simulink model "SolarInverter_DigitalTwin"  (R2019b)
settings: Solver=ode23tb  StartTime=0.0  StopTime=inf  RelTol=1e-3
InitFcn:
  | SolarInverter_Params();
values from neighbouring files (symbols this model uses):
  Fnom = 60    [SolarInverter_Params.m]
  Pnom = 112e3    (= 112000)    [SolarInverter_Params.m]
  reec_dbd1 = -0.1    [SolarInverter_Params.m]
  reec_dbd2 = 0.1    [SolarInverter_Params.m]
  reec_dPmax = 0.1    [SolarInverter_Params.m]
  reec_dPmin = -0.1    [SolarInverter_Params.m]
  reec_Imax = 1    [SolarInverter_Params.m]
  reec_Iqhl = 1.0    (= 1)    [SolarInverter_Params.m]
  reec_Iqll = -0.4    [SolarInverter_Params.m]
  reec_Kqi = 0.0    (= 0)    [SolarInverter_Params.m]
  reec_Kqp = 0    [SolarInverter_Params.m]
  reec_Kvi = 0.0    (= 0)    [SolarInverter_Params.m]
  reec_Kvp = 0.1    [SolarInverter_Params.m]
  reec_Pmax = 1.0    (= 1)    [SolarInverter_Params.m]
  reec_Pmin = 0    [SolarInverter_Params.m]
  reec_Qmax = 0.435    [SolarInverter_Params.m]
  reec_Qmin = -0.435    [SolarInverter_Params.m]
  reec_Tiq = 0.02    [SolarInverter_Params.m]
  reec_Tp = 0.02    [SolarInverter_Params.m]
  reec_Tpord = 0.1    [SolarInverter_Params.m]
  reec_Trv = 0.01    [SolarInverter_Params.m]
  reec_Vdip = 0.9    [SolarInverter_Params.m]
  reec_Vmax = 1.10    (= 1.1)    [SolarInverter_Params.m]
  reec_Vmin = 0.9    [SolarInverter_Params.m]
  reec_Vup = 1.15    [SolarInverter_Params.m]
  regc_Brkpt = 0.9    [SolarInverter_Params.m]
  regc_Iolim = -1.2    [SolarInverter_Params.m]
  regc_Iqrmax = 999.9    [SolarInverter_Params.m]
  regc_Iqrmin = -999.9    [SolarInverter_Params.m]
  regc_Ivpnt0 = 0.4    [SolarInverter_Params.m]
  regc_Ivpnt1 = 0.8    [SolarInverter_Params.m]
  regc_Khv = 0.0    (= 0)    [SolarInverter_Params.m]
  regc_Lvpl1 = 1.0    (= 1)    [SolarInverter_Params.m]
  regc_Lvplsw = 0    [SolarInverter_Params.m]
  regc_rrpwr = 10    [SolarInverter_Params.m]
  regc_Tfltr = 0.02    [SolarInverter_Params.m]
  regc_Tg = 0.1    [SolarInverter_Params.m]
  regc_Volim = 1.1    [SolarInverter_Params.m]
  regc_Zerox = 0.5    [SolarInverter_Params.m]
  repc_db1 = 0    [SolarInverter_Params.m]
  repc_Ddn = 20    [SolarInverter_Params.m]
  repc_Dup = 0    [SolarInverter_Params.m]
  repc_emax = 999    [SolarInverter_Params.m]
  repc_emin = -999    [SolarInverter_Params.m]
  repc_fdbd1 = 0.01*0    (= 0)    [SolarInverter_Params.m]
  repc_fdbd2 = -0.01*0    (= 0)    [SolarInverter_Params.m]
  repc_femax = 999    [SolarInverter_Params.m]
  repc_femin = -999    [SolarInverter_Params.m]
  repc_Kc = 0.05    [SolarInverter_Params.m]
  repc_Ki = 1.8    [SolarInverter_Params.m]
  repc_Kig = 0.5    [SolarInverter_Params.m]
  repc_Kp = 0.6    [SolarInverter_Params.m]
  repc_Kpg = 0.1    [SolarInverter_Params.m]
  repc_Pmax = 1    [SolarInverter_Params.m]
  repc_Pmin = 0    [SolarInverter_Params.m]
  repc_Qmax = inf    [SolarInverter_Params.m]
  repc_Qmin = -inf    [SolarInverter_Params.m]
  repc_Rc = 0    [SolarInverter_Params.m]
  repc_Tfltr = 0.02    [SolarInverter_Params.m]
  repc_Tft = 0.5    [SolarInverter_Params.m]
  repc_Tfv = 0.8    [SolarInverter_Params.m]
  repc_Tlag = 0.2    [SolarInverter_Params.m]
  repc_Tp = 0.25    [SolarInverter_Params.m]
  repc_Vfrz = 0.7    [SolarInverter_Params.m]
  repc_Xc = 0    [SolarInverter_Params.m]
  Vnom = 142e3    (= 142000)    [SolarInverter_Params.m]
undefined symbols (not defined in the file or in its folder): gcbh, j, sps_rtmsupport
libraries: simulink x15, powerlib x7, powerlib_meascontrol x2
(part 2 of 2)

== system SolarInverter_DigitalTwin/Utility-scale Solar Plant Controller/P Filter ==
  u : Inport
  1/(taus+1) : Subsystem  mask{tau=tau, vmax=vmax, vmin=vmin}
      mask prompts: tau "Time Constant"
  k : Gain  Gain=k
  y : Outport  VectorParamsAs1DForOutWhenUnconnected=off
  wires:
  k/1 -> 1/(taus+1)/1(u)
  u/1 -> k/1
  1/(taus+1)/1(y) -> y/1

== system SolarInverter_DigitalTwin/Utility-scale Solar Plant Controller/Q Filter ==
  u : Inport
  1/(taus+1) : Subsystem  mask{tau=tau, vmax=vmax, vmin=vmin}
      mask prompts: tau "Time Constant"
  k : Gain  Gain=k
  y : Outport  VectorParamsAs1DForOutWhenUnconnected=off
  wires:
  k/1 -> 1/(taus+1)/1(u)
  u/1 -> k/1
  1/(taus+1)/1(y) -> y/1

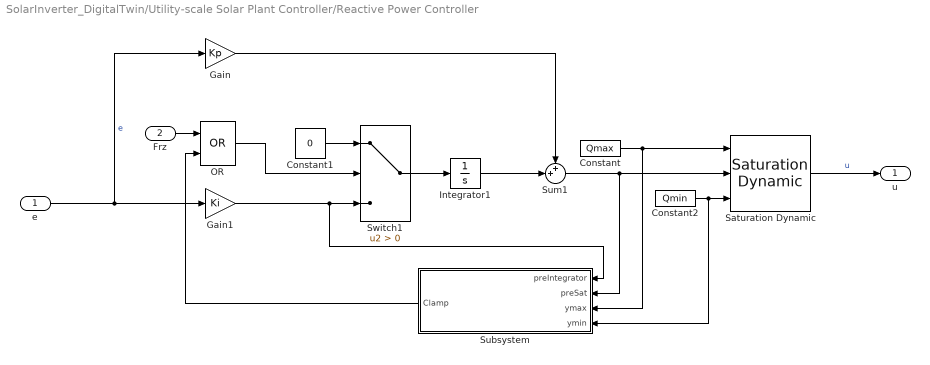
== system SolarInverter_DigitalTwin/Utility-scale Solar Plant Controller/Reactive Power Controller ==
  e : Inport
  Frz : Inport  Port=2
  Constant : Constant  Value=Qmax
  Constant1 : Constant  Value=0
  Constant2 : Constant  Value=Qmin
  Gain : Gain  Gain=Kp
  Gain1 : Gain  Gain=Ki
  Integrator1 : Integrator
  OR : Logic  Operator=OR  AllPortsSameDT=off  OutDataTypeStr=boolean
  Saturation Dynamic : simulink/Discontinuities/Saturation Dynamic  OutMin=[]  OutMax=[]  OutDataTypeStr=Inherit: Same as second input  OutDataType=fixdt(1, 16)  OutScaling=2^-10  DoSatur=off
  Subsystem : Subsystem
  Sum1 : Sum  Inputs=++|
  Switch1 : Switch  Criteria=u2 > Threshold
  u : Outport  VectorParamsAs1DForOutWhenUnconnected=off
  wires:
  OR/1 -> Switch1/2
  Subsystem/1(Clamp) -> OR/2
  Frz/1 -> OR/1
  Constant2/1 -> Saturation Dynamic/3, Subsystem/4(ymin)
  Sum1/1 -> Saturation Dynamic/2, Subsystem/2(preSat)
  Saturation Dynamic/1 -> u/1  "u"
  Switch1/1 -> Integrator1/1
  Gain1/1 -> Switch1/3, Subsystem/1(preIntegrator)
  Integrator1/1 -> Sum1/2
  Constant/1 -> Saturation Dynamic/1, Subsystem/3(ymax)
  Constant1/1 -> Switch1/1
  e/1 -> Gain1/1, Gain/1  "e"
  Gain/1 -> Sum1/1

== system SolarInverter_DigitalTwin/Utility-scale Solar Plant Controller/Subsystem ==
  Ibranch : Inport
  Vreg : Inport  Port=2
  Complex to Magnitude : ComplexToMagnitudeAngle  Output=Magnitude
  Gain : Gain  Gain=Rc
  Gain1 : Gain  Gain=j*Xc
  Sum : Sum  Inputs=|++
  Sum1 : Sum  Inputs=|-+
  Ve : Outport  VectorParamsAs1DForOutWhenUnconnected=off
  wires:
  Ibranch/1 -> Gain/1, Gain1/1
  Gain/1 -> Sum/1
  Vreg/1 -> Sum1/2
  Sum/1 -> Sum1/1
  Gain1/1 -> Sum/2
  Sum1/1 -> Complex to Magnitude/1
  Complex to Magnitude/1 -> Ve/1  "Ve"

== system SolarInverter_DigitalTwin/Utility-scale Solar Plant Controller/Vcomp Filter ==
  u : Inport
  1/(taus+1) : Subsystem  mask{tau=tau, vmax=vmax, vmin=vmin}
      mask prompts: tau "Time Constant"
  k : Gain  Gain=k
  y : Outport  VectorParamsAs1DForOutWhenUnconnected=off
  wires:
  k/1 -> 1/(taus+1)/1(u)
  u/1 -> k/1
  1/(taus+1)/1(y) -> y/1

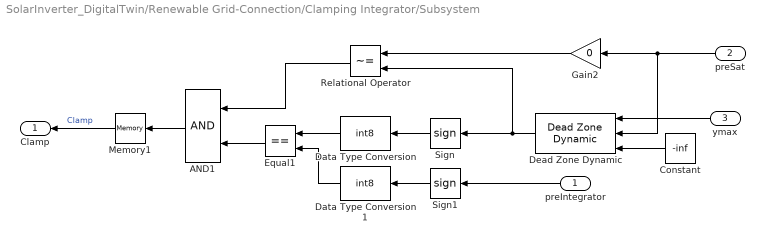
== system SolarInverter_DigitalTwin/Renewable Grid-Connection/Clamping Integrator/Subsystem ==
  preIntegrator : Inport
  preSat : Inport  Port=2
  ymax : Inport  Port=3
  AND1 : Logic  AllPortsSameDT=off  OutDataTypeStr=boolean
  Constant : Constant  Value=-inf
  Data Type Conversion : DataTypeConversion  OutDataTypeStr=int8
  Data Type Conversion1 : DataTypeConversion  OutDataTypeStr=int8
  Dead Zone Dynamic : simulink/Discontinuities/Dead Zone Dynamic
      settings: SourceProductName=Simulink  SourceProductBaseCode=SL
  Equal1 : RelationalOperator  Operator===  OutDataTypeStr=boolean  RndMeth=Simplest
  Gain2 : Gain  Gain=0
  Memory1 : Memory
  Relational Operator : RelationalOperator  Operator=~=  OutDataTypeStr=boolean  RndMeth=Simplest
  Sign : Signum
  Sign1 : Signum
  Clamp : Outport  VectorParamsAs1DForOutWhenUnconnected=off
  wires:
  Sign/1 -> Data Type Conversion/1
  AND1/1 -> Memory1/1
  Dead Zone Dynamic/1 -> Relational Operator/2, Sign/1
  Data Type Conversion/1 -> Equal1/1
  Gain2/1 -> Relational Operator/1
  Equal1/1 -> AND1/2
  preSat/1 -> Dead Zone Dynamic/2, Gain2/1
  Relational Operator/1 -> AND1/1
  Sign1/1 -> Data Type Conversion1/1
  preIntegrator/1 -> Sign1/1
  Data Type Conversion1/1 -> Equal1/2
  ymax/1 -> Dead Zone Dynamic/1
  Constant/1 -> Dead Zone Dynamic/3
  Memory1/1 -> Clamp/1  "Clamp"

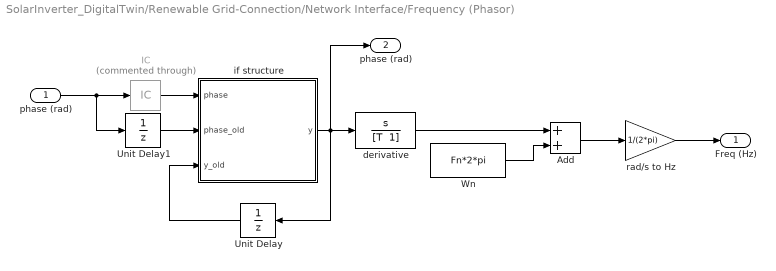
== system SolarInverter_DigitalTwin/Renewable Grid-Connection/Network Interface/Frequency (Phasor) ==
  phase (rad) : Inport
  " Wn" : Constant  Value=Fn*2*pi
  Add : Sum
  IC : InitialCondition  Commented=through  Value=0
  Unit Delay : UnitDelay  SampleTime=-1  HasFrameUpgradeWarning=on
  Unit Delay1 : UnitDelay  SampleTime=-1  HasFrameUpgradeWarning=on
  derivative : TransferFcn  Numerator="[1  0]"  Denominator="[T  1]"
  if structure : MATLAB Function  TreatAsAtomicUnit=on
  rad/s to Hz : Gain  Gain=1/(2*pi)
  Freq (Hz) : Outport  VectorParamsAs1DForOutWhenUnconnected=off
  "phase (rad) " : Outport  Port=2  VectorParamsAs1DForOutWhenUnconnected=off
  wires:
  Add/1 -> rad/s to Hz/1
  if structure/1(y) -> Unit Delay/1, derivative/1, "phase (rad) "/1
  rad/s to Hz/1 -> Freq (Hz)/1
  derivative/1 -> Add/1
  " Wn"/1 -> Add/2
  IC/1 -> if structure/1(phase)
  Unit Delay/1 -> if structure/3(y_old)
  Unit Delay1/1 -> if structure/2(phase_old)
  phase (rad)/1 -> Unit Delay1/1, IC/1

== system SolarInverter_DigitalTwin/Renewable Grid-Connection/Network Interface/Three-phase Interface ==
  Iactive : Inport
  Ireactive : Inport  Port=2
  Controlled Current Source : powerlib/Electrical Sources/Controlled Current Source  Initialize=on  Source_Type=AC  Amplitude=-1*Pnom/sqrt(3)/Vnom*sqrt(2)  Phase=0  Frequency=Fnom  Measurements=None
      settings: SourceProductName=Simscape Electrical
  Controlled Current Source1 : powerlib/Electrical Sources/Controlled Current Source  Initialize=on  Source_Type=AC  Amplitude=-1*Pnom/sqrt(3)/Vnom*sqrt(2)  Phase=120  Frequency=Fnom  Measurements=None
      settings: SourceProductName=Simscape Electrical
  Gain : Gain  Gain=exp(-j*2*pi/3)
  Real-Imag to Complex : RealImagToComplex
  "pu->A " : Gain  Gain=Pnom/sqrt(3)/Vnom*sqrt(2)  SaturateOnIntegerOverflow=on  OutDataTypeStr=Inherit: Same as input  ParamDataTypeStr=Inherit: Same as input
  pu->A 1 : Gain  Gain=Pnom/sqrt(3)/Vnom*sqrt(2)  SaturateOnIntegerOverflow=on  OutDataTypeStr=Inherit: Same as input  ParamDataTypeStr=Inherit: Same as input
  A : PMIOPort  Side=Right
  B : PMIOPort  Port=2  Side=Right
  C : PMIOPort  Port=3  Side=Right
  wires:
  pu->A 1/1 -> Controlled Current Source1/1
  Gain/1 -> pu->A 1/1  "Ib"
  Real-Imag to Complex/1 -> Gain/1, "pu->A "/1  "Ia"
  "pu->A "/1 -> Controlled Current Source/1
  Iactive/1 -> Real-Imag to Complex/1
  Ireactive/1 -> Real-Imag to Complex/2
  connections:
  Controlled Current Source/RConn1 -- C/RConn1 -- Controlled Current Source1/RConn1
  A/RConn1 -- Controlled Current Source/LConn1
  B/RConn1 -- Controlled Current Source1/LConn1

== system SolarInverter_DigitalTwin/Renewable Grid-Connection/Q Current Filter/1//(taus+1) ==
  note: disable integrator and pass through signal if tau is zero
  u : Inport
  Constant : Constant  Value=tau
  Gain1 : Gain  Gain=1/(tau+eps)  SaturateOnIntegerOverflow=on  OutDataTypeStr=Inherit: Same as input  ParamDataTypeStr=Inherit: Same as input
  Integrator : Integrator  LimitOutput=on  UpperSaturationLimit=vmax  LowerSaturationLimit=vmin
  Sum : Sum  Inputs=|+-  SaturateOnIntegerOverflow=on  InputSameDT=on  OutDataTypeStr=Inherit: Same as first input
  Switch : Switch  Criteria=u2 > Threshold
  Switch1 : Switch  Criteria=u2 > Threshold
  y : Outport  VectorParamsAs1DForOutWhenUnconnected=off
  wires:
  Switch1/1 -> y/1
  Switch/1 -> Integrator/1
  Gain1/1 -> Switch/1
  Constant/1 -> Switch/2, Switch1/2, Switch/3
  Integrator/1 -> Switch1/1, Sum/2
  Sum/1 -> Gain1/1
  u/1 -> Sum/1, Switch1/3

== system SolarInverter_DigitalTwin/Renewable Grid-Connection/Voltage Filter/1//(taus+1) ==
  note: disable integrator and pass through signal if tau is zero
  u : Inport
  Constant : Constant  Value=tau
  Gain1 : Gain  Gain=1/(tau+eps)  SaturateOnIntegerOverflow=on  OutDataTypeStr=Inherit: Same as input  ParamDataTypeStr=Inherit: Same as input
  Integrator : Integrator  InitialCondition=1  LimitOutput=on  UpperSaturationLimit=vmax  LowerSaturationLimit=vmin
  Sum : Sum  Inputs=|+-  SaturateOnIntegerOverflow=on  InputSameDT=on  OutDataTypeStr=Inherit: Same as first input
  Switch : Switch  Criteria=u2 > Threshold
  Switch1 : Switch  Criteria=u2 > Threshold
  y : Outport  VectorParamsAs1DForOutWhenUnconnected=off
  wires:
  Sum/1 -> Gain1/1
  Integrator/1 -> Sum/2, Switch1/1
  Constant/1 -> Switch/3, Switch1/2, Switch/2
  Gain1/1 -> Switch/1
  Switch/1 -> Integrator/1
  Switch1/1 -> y/1
  u/1 -> Switch1/3, Sum/1

== system SolarInverter_DigitalTwin/Utility-scale Solar Electrical Controller/Active Power Filter/1//(taus+1) ==
  note: disable integrator and pass through signal if tau is zero
  u : Inport
  Constant : Constant  Value=tau
  Gain1 : Gain  Gain=1/(tau+eps)  SaturateOnIntegerOverflow=on  OutDataTypeStr=Inherit: Same as input  ParamDataTypeStr=Inherit: Same as input
  Integrator : Integrator  InitialCondition=1  LimitOutput=on  UpperSaturationLimit=vmax  LowerSaturationLimit=vmin
  Sum : Sum  Inputs=|+-  SaturateOnIntegerOverflow=on  InputSameDT=on  OutDataTypeStr=Inherit: Same as first input
  Switch : Switch  Criteria=u2 > Threshold
  Switch1 : Switch  Criteria=u2 > Threshold
  y : Outport  VectorParamsAs1DForOutWhenUnconnected=off
  wires:
  u/1 -> Switch1/3, Sum/1
  Sum/1 -> Gain1/1
  Integrator/1 -> Sum/2, Switch1/1
  Constant/1 -> Switch/3, Switch1/2, Switch/2
  Gain1/1 -> Switch/1
  Switch/1 -> Integrator/1
  Switch1/1 -> y/1

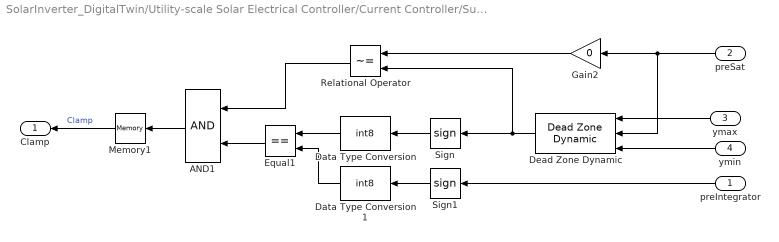
== system SolarInverter_DigitalTwin/Utility-scale Solar Electrical Controller/Current Controller/Subsystem ==
  preIntegrator : Inport
  preSat : Inport  Port=2
  ymax : Inport  Port=3
  ymin : Inport  Port=4
  AND1 : Logic  AllPortsSameDT=off  OutDataTypeStr=boolean
  Data Type Conversion : DataTypeConversion  OutDataTypeStr=int8
  Data Type Conversion1 : DataTypeConversion  OutDataTypeStr=int8
  Dead Zone Dynamic : simulink/Discontinuities/Dead Zone Dynamic
      settings: SourceProductName=Simulink  SourceProductBaseCode=SL
  Equal1 : RelationalOperator  Operator===  OutDataTypeStr=boolean  RndMeth=Simplest
  Gain2 : Gain  Gain=0
  Memory1 : Memory
  Relational Operator : RelationalOperator  Operator=~=  OutDataTypeStr=boolean  RndMeth=Simplest
  Sign : Signum
  Sign1 : Signum
  Clamp : Outport  VectorParamsAs1DForOutWhenUnconnected=off
  wires:
  Sign/1 -> Data Type Conversion/1
  AND1/1 -> Memory1/1
  Dead Zone Dynamic/1 -> Relational Operator/2, Sign/1
  Data Type Conversion/1 -> Equal1/1
  Gain2/1 -> Relational Operator/1
  Equal1/1 -> AND1/2
  preSat/1 -> Dead Zone Dynamic/2, Gain2/1
  Relational Operator/1 -> AND1/1
  Sign1/1 -> Data Type Conversion1/1
  preIntegrator/1 -> Sign1/1
  Data Type Conversion1/1 -> Equal1/2
  ymax/1 -> Dead Zone Dynamic/1
  ymin/1 -> Dead Zone Dynamic/3
  Memory1/1 -> Clamp/1  "Clamp"

== system SolarInverter_DigitalTwin/Utility-scale Solar Electrical Controller/Current Filter/1//(taus+1) ==
  note: disable integrator and pass through signal if tau is zero
  u : Inport
  Vflag : Inport  Port=2
  Constant : Constant  Value=tau
  Constant1 : Constant  Value=0
  Gain1 : Gain  Gain=1/(tau+eps)  SaturateOnIntegerOverflow=on  OutDataTypeStr=Inherit: Same as input  ParamDataTypeStr=Inherit: Same as input
  Integrator : Integrator  LimitOutput=on  UpperSaturationLimit=vmax  LowerSaturationLimit=vmin
  Subsystem : Subsystem
  Sum : Sum  Inputs=|+-  SaturateOnIntegerOverflow=on  InputSameDT=on  OutDataTypeStr=Inherit: Same as first input
  Switch : Switch  Criteria=u2 > Threshold
  Switch1 : Switch  Criteria=u2 > Threshold
  y : Outport  VectorParamsAs1DForOutWhenUnconnected=off
  wires:
  Switch1/1 -> y/1
  Switch/1 -> Integrator/1
  Gain1/1 -> Switch/1
  Constant/1 -> Switch1/2, Subsystem/1(tau)
  Integrator/1 -> Switch1/1, Sum/2
  Sum/1 -> Gain1/1
  u/1 -> Sum/1, Switch1/3
  Constant1/1 -> Switch/3
  Subsystem/1(Out1) -> Switch/2
  Vflag/1 -> Subsystem/2(Vflag)

== system SolarInverter_DigitalTwin/Utility-scale Solar Electrical Controller/Reference Power Filter/1//(taus+1) ==
  note: disable integrator and pass through signal if tau is zero
  u : Inport
  Vflag : Inport  Port=2
  Constant : Constant  Value=tau
  Constant1 : Constant  Value=0
  Gain1 : Gain  Gain=1/(tau+eps)  SaturateOnIntegerOverflow=on  OutDataTypeStr=Inherit: Same as input  ParamDataTypeStr=Inherit: Same as input
  Integrator : Integrator  InitialCondition=0.999  LimitOutput=on  UpperSaturationLimit=vmax  LowerSaturationLimit=vmin
  Subsystem : Subsystem
  Sum : Sum  Inputs=|+-  SaturateOnIntegerOverflow=on  InputSameDT=on  OutDataTypeStr=Inherit: Same as first input
  Switch : Switch  Criteria=u2 > Threshold
  Switch1 : Switch  Criteria=u2 > Threshold
  y : Outport  VectorParamsAs1DForOutWhenUnconnected=off
  wires:
  Vflag/1 -> Subsystem/2(Vflag)
  Subsystem/1(Out1) -> Switch/2
  Constant1/1 -> Switch/3
  u/1 -> Switch1/3, Sum/1
  Sum/1 -> Gain1/1
  Integrator/1 -> Sum/2, Switch1/1
  Constant/1 -> Subsystem/1(tau), Switch1/2
  Gain1/1 -> Switch/1
  Switch/1 -> Integrator/1
  Switch1/1 -> y/1

== system SolarInverter_DigitalTwin/Utility-scale Solar Electrical Controller/Vt Filter/1//(taus+1) ==
  note: disable integrator and pass through signal if tau is zero
  u : Inport
  Constant : Constant  Value=tau
  Gain1 : Gain  Gain=1/(tau+eps)  SaturateOnIntegerOverflow=on  OutDataTypeStr=Inherit: Same as input  ParamDataTypeStr=Inherit: Same as input
  Integrator : Integrator  InitialCondition=1  LimitOutput=on  UpperSaturationLimit=vmax  LowerSaturationLimit=vmin
  Sum : Sum  Inputs=|+-  SaturateOnIntegerOverflow=on  InputSameDT=on  OutDataTypeStr=Inherit: Same as first input
  Switch : Switch  Criteria=u2 > Threshold
  Switch1 : Switch  Criteria=u2 > Threshold
  y : Outport  VectorParamsAs1DForOutWhenUnconnected=off
  wires:
  u/1 -> Switch1/3, Sum/1
  Sum/1 -> Gain1/1
  Integrator/1 -> Sum/2, Switch1/1
  Constant/1 -> Switch/3, Switch1/2, Switch/2
  Gain1/1 -> Switch/1
  Switch/1 -> Integrator/1
  Switch1/1 -> y/1

== system SolarInverter_DigitalTwin/Utility-scale Solar Plant Controller/Lag Filter/1//(taus+1) ==
  note: disable integrator and pass through signal if tau is zero
  u : Inport
  Constant : Constant  Value=tau
  Gain1 : Gain  Gain=1/(tau+eps)  SaturateOnIntegerOverflow=on  OutDataTypeStr=Inherit: Same as input  ParamDataTypeStr=Inherit: Same as input
  Integrator : Integrator  InitialCondition=1  LimitOutput=on  UpperSaturationLimit=vmax  LowerSaturationLimit=vmin
  Sum : Sum  Inputs=|+-  SaturateOnIntegerOverflow=on  InputSameDT=on  OutDataTypeStr=Inherit: Same as first input
  Switch : Switch  Criteria=u2 > Threshold
  Switch1 : Switch  Criteria=u2 > Threshold
  y : Outport  VectorParamsAs1DForOutWhenUnconnected=off
  wires:
  u/1 -> Switch1/3, Sum/1
  Sum/1 -> Gain1/1
  Integrator/1 -> Sum/2, Switch1/1
  Constant/1 -> Switch/3, Switch1/2, Switch/2
  Gain1/1 -> Switch/1
  Switch/1 -> Integrator/1
  Switch1/1 -> y/1

== system SolarInverter_DigitalTwin/Utility-scale Solar Plant Controller/P Filter/1//(taus+1) ==
  note: disable integrator and pass through signal if tau is zero
  u : Inport
  Constant : Constant  Value=tau
  Gain1 : Gain  Gain=1/(tau+eps)  SaturateOnIntegerOverflow=on  OutDataTypeStr=Inherit: Same as input  ParamDataTypeStr=Inherit: Same as input
  Integrator : Integrator  InitialCondition=1  LimitOutput=on  UpperSaturationLimit=vmax  LowerSaturationLimit=vmin
  Sum : Sum  Inputs=|+-  SaturateOnIntegerOverflow=on  InputSameDT=on  OutDataTypeStr=Inherit: Same as first input
  Switch : Switch  Criteria=u2 > Threshold
  Switch1 : Switch  Criteria=u2 > Threshold
  y : Outport  VectorParamsAs1DForOutWhenUnconnected=off
  wires:
  u/1 -> Switch1/3, Sum/1
  Sum/1 -> Gain1/1
  Integrator/1 -> Sum/2, Switch1/1
  Constant/1 -> Switch/3, Switch1/2, Switch/2
  Gain1/1 -> Switch/1
  Switch/1 -> Integrator/1
  Switch1/1 -> y/1

== system SolarInverter_DigitalTwin/Utility-scale Solar Plant Controller/Q Filter/1//(taus+1) ==
  note: disable integrator and pass through signal if tau is zero
  u : Inport
  Constant : Constant  Value=tau
  Gain1 : Gain  Gain=1/(tau+eps)  SaturateOnIntegerOverflow=on  OutDataTypeStr=Inherit: Same as input  ParamDataTypeStr=Inherit: Same as input
  Integrator : Integrator  LimitOutput=on  UpperSaturationLimit=vmax  LowerSaturationLimit=vmin
  Sum : Sum  Inputs=|+-  SaturateOnIntegerOverflow=on  InputSameDT=on  OutDataTypeStr=Inherit: Same as first input
  Switch : Switch  Criteria=u2 > Threshold
  Switch1 : Switch  Criteria=u2 > Threshold
  y : Outport  VectorParamsAs1DForOutWhenUnconnected=off
  wires:
  u/1 -> Switch1/3, Sum/1
  Sum/1 -> Gain1/1
  Integrator/1 -> Sum/2, Switch1/1
  Constant/1 -> Switch/3, Switch1/2, Switch/2
  Gain1/1 -> Switch/1
  Switch/1 -> Integrator/1
  Switch1/1 -> y/1

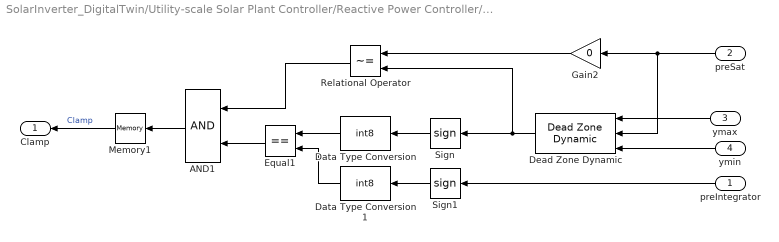
== system SolarInverter_DigitalTwin/Utility-scale Solar Plant Controller/Reactive Power Controller/Subsystem ==
  preIntegrator : Inport
  preSat : Inport  Port=2
  ymax : Inport  Port=3
  ymin : Inport  Port=4
  AND1 : Logic  AllPortsSameDT=off  OutDataTypeStr=boolean
  Data Type Conversion : DataTypeConversion  OutDataTypeStr=int8
  Data Type Conversion1 : DataTypeConversion  OutDataTypeStr=int8
  Dead Zone Dynamic : simulink/Discontinuities/Dead Zone Dynamic
      settings: SourceProductName=Simulink  SourceProductBaseCode=SL
  Equal1 : RelationalOperator  Operator===  OutDataTypeStr=boolean  RndMeth=Simplest
  Gain2 : Gain  Gain=0
  Memory1 : Memory
  Relational Operator : RelationalOperator  Operator=~=  OutDataTypeStr=boolean  RndMeth=Simplest
  Sign : Signum
  Sign1 : Signum
  Clamp : Outport  VectorParamsAs1DForOutWhenUnconnected=off
  wires:
  Memory1/1 -> Clamp/1  "Clamp"
  ymin/1 -> Dead Zone Dynamic/3
  ymax/1 -> Dead Zone Dynamic/1
  Data Type Conversion1/1 -> Equal1/2
  preIntegrator/1 -> Sign1/1
  Sign1/1 -> Data Type Conversion1/1
  Relational Operator/1 -> AND1/1
  preSat/1 -> Gain2/1, Dead Zone Dynamic/2
  Equal1/1 -> AND1/2
  Gain2/1 -> Relational Operator/1
  Data Type Conversion/1 -> Equal1/1
  Dead Zone Dynamic/1 -> Sign/1, Relational Operator/2
  AND1/1 -> Memory1/1
  Sign/1 -> Data Type Conversion/1

== system SolarInverter_DigitalTwin/Utility-scale Solar Plant Controller/Vcomp Filter/1//(taus+1) ==
  note: disable integrator and pass through signal if tau is zero
  u : Inport
  Constant : Constant  Value=tau
  Gain1 : Gain  Gain=1/(tau+eps)  SaturateOnIntegerOverflow=on  OutDataTypeStr=Inherit: Same as input  ParamDataTypeStr=Inherit: Same as input
  Integrator : Integrator  InitialCondition=1  LimitOutput=on  UpperSaturationLimit=vmax  LowerSaturationLimit=vmin
  Sum : Sum  Inputs=|+-  SaturateOnIntegerOverflow=on  InputSameDT=on  OutDataTypeStr=Inherit: Same as first input
  Switch : Switch  Criteria=u2 > Threshold
  Switch1 : Switch  Criteria=u2 > Threshold
  y : Outport  VectorParamsAs1DForOutWhenUnconnected=off
  wires:
  u/1 -> Switch1/3, Sum/1
  Sum/1 -> Gain1/1
  Integrator/1 -> Sum/2, Switch1/1
  Constant/1 -> Switch/3, Switch1/2, Switch/2
  Gain1/1 -> Switch/1
  Switch/1 -> Integrator/1
  Switch1/1 -> y/1

== system SolarInverter_DigitalTwin/Utility-scale Solar Electrical Controller/Current Filter/1//(taus+1)/Subsystem ==
  tau : Inport
  Vflag : Inport  Port=2
  AND : Logic  AllPortsSameDT=off  OutDataTypeStr=boolean
  Compare To Zero : simulink/Logic and Bit Operations/Compare To Zero  relop=>  OutDataTypeStr=boolean
  NOT : Logic  Operator=NOT  AllPortsSameDT=off  OutDataTypeStr=boolean
  Out1 : Outport  VectorParamsAs1DForOutWhenUnconnected=off
  wires:
  NOT/1 -> AND/2
  tau/1 -> Compare To Zero/1
  AND/1 -> Out1/1
  Compare To Zero/1 -> AND/1
  Vflag/1 -> NOT/1

== system SolarInverter_DigitalTwin/Utility-scale Solar Electrical Controller/Reference Power Filter/1//(taus+1)/Subsystem ==
  tau : Inport
  Vflag : Inport  Port=2
  AND : Logic  AllPortsSameDT=off  OutDataTypeStr=boolean
  Compare To Zero : simulink/Logic and Bit Operations/Compare To Zero  relop=>  OutDataTypeStr=boolean
  NOT : Logic  Operator=NOT  AllPortsSameDT=off  OutDataTypeStr=boolean
  Out1 : Outport  VectorParamsAs1DForOutWhenUnconnected=off
  wires:
  Vflag/1 -> NOT/1
  Compare To Zero/1 -> AND/1
  AND/1 -> Out1/1
  tau/1 -> Compare To Zero/1
  NOT/1 -> AND/2

== stateflow chart SolarInverter_DigitalTwin/Local and Plant Level Controller ==
  state ReactivePower [parallel]
    Mode.VcompFlag = 1;
    settings: executionOrder=1
    state V_Control
      Mode.PfFlag = 0;
      state PlantLevel
        Mode.QFlag = 0;
        Mode.RefFlag = 1;
      state LocalLevel
        Mode.VFlag = 0;
        Mode.QFlag = 1;
      (default) -> ReactivePower.V_Control.PlantLevel
      ReactivePower.V_Control.LocalLevel -> ReactivePower.V_Control.PlantLevel : [PlantControl == 1]
      ReactivePower.V_Control.PlantLevel -> ReactivePower.V_Control.LocalLevel : [PlantControl == 0]
    state Q_Control
      Mode.PfFlag = 0;
      Mode.VFlag = 1;
      state PlantLevel
        Mode.QFlag = 0;
        Mode.RefFlag = 0;
      state LocalLevel
        Mode.QFlag = 0;
      (default) -> ReactivePower.Q_Control.PlantLevel
      ReactivePower.Q_Control.LocalLevel -> ReactivePower.Q_Control.PlantLevel : [PlantControl == 1]
      ReactivePower.Q_Control.PlantLevel -> ReactivePower.Q_Control.LocalLevel : [PlantControl == 0]
    state PowerFactor
      Mode.PfFlag = 1;
      Mode.QFlag = 0;
    (default) -> V_Control
    Q_Control -> V_Control [order 1] : [QControl == 0]
    V_Control -> Q_Control [order 1] : [QControl == 1]
    PowerFactor -> Q_Control [order 2] : [PFControl == 0 && ...
        | QControl == 1]
    Q_Control -> PowerFactor [order 2] : [PFControl == 1]
    PowerFactor -> V_Control [order 1] : [PFControl == 0 && ...
        | QControl == 0]
    V_Control -> PowerFactor [order 2] : [PFControl == 1]
  state ActivePower [parallel]
    settings: executionOrder=2
    state NoGovenorResponse
      Mode.FrqFlag = 0;
    state GovernorResponse
      Mode.FrqFlag = 1;
    (default) -> GovernorResponse
    GovernorResponse -> NoGovenorResponse : [FrqControl == 0]
    NoGovenorResponse -> GovernorResponse : [FrqControl == 1]
  state CoordinatedQV [parallel]
    settings: executionOrder=3
    state QVControl_Off
      Mode.VFlag = 0;
    state QVControl_On
      Mode.VFlag = 1;
    (default) -> QVControl_Off
    QVControl_Off -> QVControl_On : [QVControl == 1 && PFControl == 0]
    QVControl_On -> QVControl_Off : [QVControl == 0]
  state PorQ_Priority [parallel]
    settings: executionOrder=4
    state Q_Priority
      Mode.PqFlag = 0;
    state P_Priority
      Mode.PqFlag = 1;
    (default) -> P_Priority
    P_Priority -> Q_Priority : [PQPriority == 0 || QControl == 1]
    Q_Priority -> P_Priority : [PQPriority == 1 && QControl == 0]
  data: QControl input; QVControl input; PFControl input; FrqControl input; PlantControl input; PQPriority input; Mode output Bus: Mode

== matlab function SolarInverter_DigitalTwin/Renewable Grid-Connection/Network Interface/Frequency (Phasor)/if structure ==
  data: phase input; phase_old input; y output; y_old input
function y = fcn(phase,phase_old,y_old)

u = phase-phase_old;
if u > 0.9*2*pi
    y=y_old+u-(2*pi);
elseif u < -(0.9*2*pi)
    y=y_old+u+(2*pi);
else
    y=y_old+u(1);
end
